simulink model "gm_cuadratico"  (R2017a)
settings: Solver=FixedStepDiscrete  StartTime=0.0  StopTime=10.0  FixedStep=0.001  RelTol=1e-3
undefined symbols (not defined in the file or in its folder): N
libraries: simulink x1
settings Model: Creator=Windows  LastModifiedBy=Windows
settings DataIOCC: LimitDataPoints=on  SaveOutput=off  SaveTime=off
settings OptimizationCC: BlockReduction=off  ConditionallyExecuteInputs=off  DefaultParameterBehavior=Inlined  LifeSpan=inf
settings DebuggingCC: AlgebraicLoopMsg=error  InheritedTsInSrcMsg=none  SingleTaskRateTransMsg=error  AllowSymbolicDim=off  StrictBusMsg=ErrorOnBusTreatedAsVector  SFUnexpectedBacktrackingDiag=warning  SFNoUnconditionalDefaultTransitionDiag=warning  SFExecutionAtInitializationDiag=none
settings HardwareCC: ProdBitPerPointer=32  ProdBitPerSizeT=32  ProdBitPerPtrDiffT=32  ProdLargestAtomicFloat=None  ProdIntDivRoundTo=Undefined  ProdEndianess=Unspecified  ProdWordSize=32  ProdHWDeviceType=ASIC/FPGA->ASIC/FPGA  ProdEqTarget=off
settings GRTTargetCC: TargetLangStandard=C89/C90 (ANSI)  GeneratePreprocessorConditionals=Disable all
settings ConfigComp: CovScope=ReferencedModels  CovMetricSettings=dw  CovHtmlReporting=on  CovSaveCumulativeToWorkspaceVar=on  CovSaveSingleToWorkspaceVar=on  CovExternalEMLEnable=off  CovSFcnEnable=off

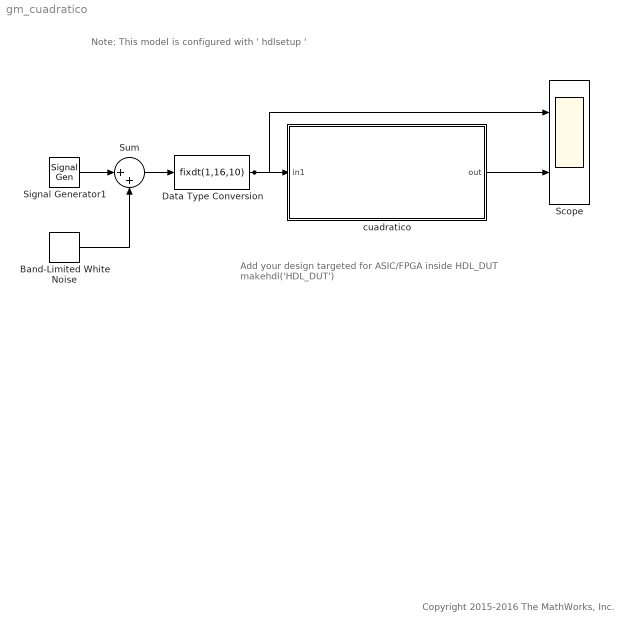
== system gm_cuadratico ==
  note: Copyright 2015-2016 The MathWorks, Inc.
  note: Add your design targeted for ASIC/FPGA inside HDL_DUT
      | makehdl('HDL_DUT')
  note: Note: This model is configured with ' hdlsetup '
  Band-Limited White Noise : simulink/Sources/Band-Limited White Noise  Cov=[0.001]  Ts=0.001  seed=[23341]
  Data Type Conversion : DataTypeConversion  OutDataTypeStr=fixdt(1,16,10)
  Scope : Scope  NumInputPorts=2
  Signal Generator1 : SignalGenerator  Frequency=2000
  Sum : Sum  Inputs=|++
  cuadratico : Subsystem
  wires:
  cuadratico/1(out) -> Scope/2
  Signal Generator1/1 -> Sum/1
  Data Type Conversion/1 -> cuadratico/1(in1), Scope/1
  Band-Limited White Noise/1 -> Sum/2
  Sum/1 -> Data Type Conversion/1

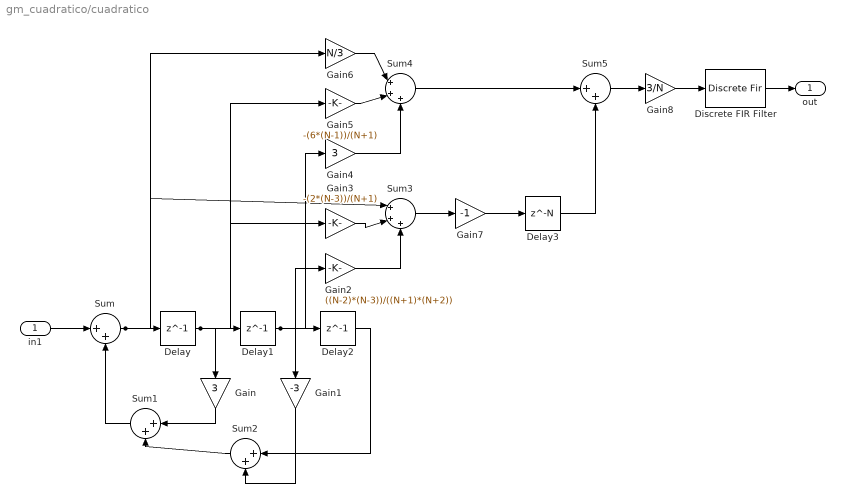
== system gm_cuadratico/cuadratico ==
  in1 : Inport  OutDataTypeStr=fixdt(1, 16, 10)  SampleTime=0
  Delay : Delay  DelayLength=1
  Delay1 : Delay  DelayLength=1
  Delay2 : Delay  DelayLength=1
  Delay3 : Delay  DelayLength=N
  Discrete FIR Filter : DiscreteFir  Coefficients=[0.2298 0.2098 0.1791 0.1557 0.1355 0.1127 0.0931 0.0749 0.0579 0.0422 0.0277 0.0146 0.0028 -0.0077 -0.0169 -0.0249 -0.0316 -0.0370 -0.0411 -0.0440 -0.0455 -0.0458 -0.0447 -0.0424 -0.0388 -0.0339 -0.0277 -0.0203 -0.0115 -0.0015 0.0097 0.0223 0.0362 0.0514 0.0679]  CoefDataTypeStr=fixdt(1,16,10)  ProductDataTypeStr=fixdt(1,16,10)  AccumDataTypeStr=fixdt(1,16,10)  OutDataTypeStr=fixdt(1,16,10)
  Gain : Gain  Gain=3
  Gain1 : Gain  Gain=-3
  Gain2 : Gain  Gain=((N-2)*(N-3))/((N+1)*(N+2))
  Gain3 : Gain  Gain=-(2*(N-3))/(N+1)
  Gain4 : Gain  Gain=3
  Gain5 : Gain  Gain=-(6*(N-1))/(N+1)
  Gain6 : Gain  Gain=N/3
  Gain7 : Gain  Gain=-1
  Gain8 : Gain  Gain=3/N
  Sum{,1..2,5} (4 alike) : Sum  Inputs=|++  AccumDataTypeStr=fixdt(1,16,10)  OutDataTypeStr=fixdt(1,16,10)
  Sum3 : Sum  Inputs=|+++  AccumDataTypeStr=fixdt(1,16,10)  OutDataTypeStr=fixdt(1,16,10)
  Sum4 : Sum  Inputs=|+++  AccumDataTypeStr=fixdt(1,16,10)  OutDataTypeStr=fixdt(1,16,10)
  out : Outport  OutDataTypeStr=fixdt(1,16,10)
  wires:
  in1/1 -> Sum/1
  Delay/1 -> Gain5/1, Gain3/1, Gain/1, Delay1/1
  Delay1/1 -> Gain4/1, Gain2/1, Gain1/1, Delay2/1
  Delay2/1 -> Sum2/1
  Delay3/1 -> Sum5/2
  Discrete FIR Filter/1 -> out/1
  Gain/1 -> Sum1/1
  Gain1/1 -> Sum2/2
  Gain2/1 -> Sum3/3
  Gain3/1 -> Sum3/2
  Gain4/1 -> Sum4/3
  Gain5/1 -> Sum4/2
  Gain6/1 -> Sum4/1
  Gain7/1 -> Delay3/1
  Gain8/1 -> Discrete FIR Filter/1
  Sum/1 -> Sum3/1, Gain6/1, Delay/1
  Sum1/1 -> Sum/2
  Sum2/1 -> Sum1/2
  Sum3/1 -> Gain7/1
  Sum4/1 -> Sum5/1
  Sum5/1 -> Gain8/1
